simulink model "BME331Lab2SimModel"  (R2023a)
settings: Solver=VariableStepAuto  StartTime=0.0  StopTime=10.0  RelTol=1e-3
model workspace (MAT data in the model file):
  Ap = Simulink.Parameter
  Ap.DataType = 'auto'
  Ap.Complexity = 'real'
  Ap.Dimensions = [0 0]
  As = Simulink.Parameter
  As.DataType = 'auto'
  As.Complexity = 'real'
  As.Dimensions = [0 0]
  Kp = Simulink.Parameter
  Kp.DataType = 'auto'
  Kp.Complexity = 'real'
  Kp.Dimensions = [0 0]
  Ks = Simulink.Parameter
  Ks.DataType = 'auto'
  Ks.Complexity = 'real'
  Ks.Dimensions = [0 0]
  fp = Simulink.Parameter
  fp.DataType = 'auto'
  fp.Complexity = 'real'
  fp.Dimensions = [0 0]
  fs = Simulink.Parameter
  fs.DataType = 'auto'
  fs.Complexity = 'real'
  fs.Dimensions = [0 0]
  s = Simulink.Parameter
  s.DataType = 'auto'
  s.Complexity = 'real'
  s.Dimensions = [0 0]
libraries: simulink x1
settings Model: Creator=ihass  LastModifiedBy=ihass

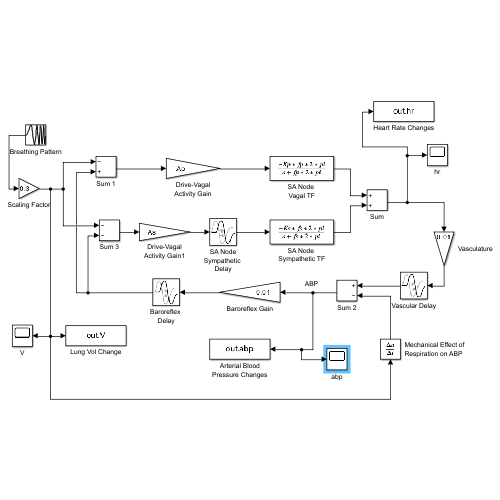
[thumbnail: Simulink's stored preview of the top-level diagram]
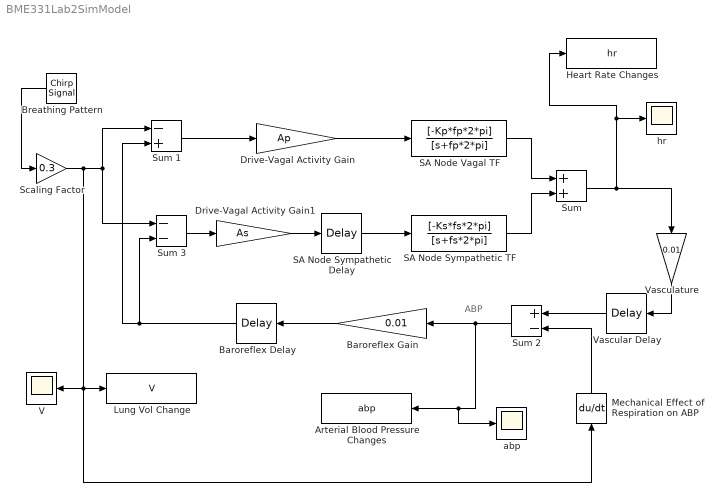
== system BME331Lab2SimModel ==
  note: ABP
  Arterial Blood Pressure Changes : ToWorkspace  VariableName=abp  SaveFormat=Timeseries  SampleTime=-1
  Baroreflex Delay : TransportDelay
  Baroreflex Gain : Gain  Gain=0.01
  Breathing Pattern : simulink/Sources/Chirp Signal  f1=0.1  T=100  f2=1
  Drive-Vagal Activity Gain : Gain  Gain=Ap
  Drive-Vagal Activity Gain1 : Gain  Gain=As
  Heart Rate Changes : ToWorkspace  VariableName=hr  SaveFormat=Timeseries  SampleTime=-1
  Lung Vol Change : ToWorkspace  VariableName=V  SaveFormat=Timeseries  SampleTime=-1
  "Mechanical Effect of Respiration on ABP " : Derivative
  SA Node Sympathetic Delay : TransportDelay
  SA Node Sympathetic TF : DiscreteTransferFcn  Numerator=[-Ks*fs*2*pi]  Denominator=[s+fs*2*pi]
  SA Node Vagal TF : DiscreteTransferFcn  Numerator=[-Kp*fp*2*pi]  Denominator=[s+fp*2*pi]
  Scaling Factor : Gain  Gain=0.3
  Sum : Sum
  Sum 1 : Sum  Inputs=-+
  Sum 2 : Sum  Inputs=+-
  Sum 3 : Sum  Inputs=--
  V : Scope
  Vascular Delay : TransportDelay
  Vasculature : Gain  Gain=0.01
  abp : Scope
  hr : Scope
  wires:
  Baroreflex Gain/1 -> Baroreflex Delay/1
  Baroreflex Delay/1 -> Sum 1/2, Sum 3/2
  Breathing Pattern/1 -> Scaling Factor/1
  Vasculature/1 -> Vascular Delay/1
  Vascular Delay/1 -> Sum 2/1
  Sum 2/1 -> abp/1, Arterial Blood Pressure Changes/1, Baroreflex Gain/1
  "Mechanical Effect of Respiration on ABP "/1 -> Sum 2/2
  Sum/1 -> Heart Rate Changes/1, hr/1, Vasculature/1
  SA Node Sympathetic Delay/1 -> SA Node Sympathetic TF/1
  SA Node Sympathetic TF/1 -> Sum/2
  SA Node Vagal TF/1 -> Sum/1
  Scaling Factor/1 -> V/1, Lung Vol Change/1, "Mechanical Effect of Respiration on ABP "/1, Sum 3/1, Sum 1/1
  Sum 1/1 -> Drive-Vagal Activity Gain/1
  Drive-Vagal Activity Gain/1 -> SA Node Vagal TF/1
  Sum 3/1 -> Drive-Vagal Activity Gain1/1
  Drive-Vagal Activity Gain1/1 -> SA Node Sympathetic Delay/1
